simulink model "Ex6_1_1_PID2"  (R2016a)
settings: Solver=VariableStepAuto  StartTime=0.0  StopTime=20  RelTol=1e-3
libraries: simulink x1
settings Model: Creator=mende  LastModifiedBy=mende

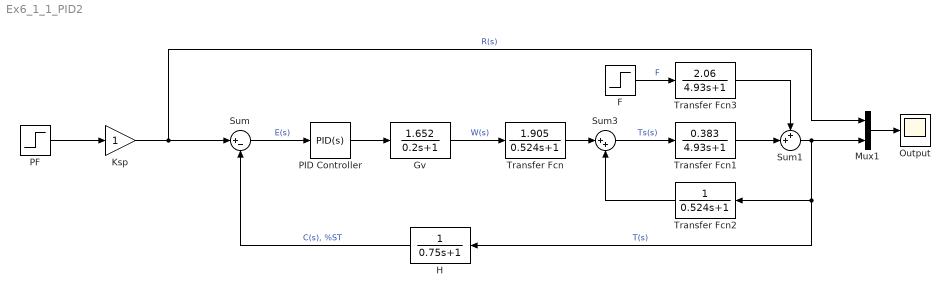
== system Ex6_1_1_PID2 ==
  F : Step  SampleTime=0
  Gv : TransferFcn  Numerator=[1.652]  Denominator=[0.2 1]
  H : TransferFcn  Denominator=[0.75 1]
  Ksp : Gain
  Mux1 : Mux  Inputs=2
  Output : Scope
  PF : Step  SampleTime=0
  PID Controller : simulink/Continuous/PID Controller  Controller=PID  TimeDomain=Continuous-time  SampleTime=-1  IntegratorMethod=Forward Euler  FilterMethod=Forward Euler  Form=Parallel  UseFilter=on  ControllerParametersSource=internal  P=6.1  I=6.1/2.3  D=6.1*0.58  N=100  InitialConditionSource=internal  InitialConditionForIntegrator=0  InitialConditionForFilter=0  ExternalReset=none  LimitOutput=off  UpperSaturationLimit=inf  LowerSaturationLimit=-inf  LinearizeAsGain=on  AntiWindupMode=none  Kb=1  TrackingMode=off  Kt=1  PParamMin=[]  PParamMax=[]  IParamMin=[]  IParamMax=[]  DParamMin=[]  DParamMax=[]  NParamMin=[]  NParamMax=[]  KbParamMin=[]  KbParamMax=[]  KtParamMin=[]  KtParamMax=[]  POutMin=[]  POutMax=[]  IOutMin=[]  IOutMax=[]  DOutMin=[]  DOutMax=[]  NOutMin=[]  NOutMax=[]  KbOutMin=[]  KbOutMax=[]  KtOutMin=[]  KtOutMax=[]  IntegratorOutMin=[]  IntegratorOutMax=[]  FilterOutMin=[]  FilterOutMax=[]  SumOutMin=[]  SumOutMax=[]  SumI1OutMin=[]  SumI1OutMax=[]  SumI2OutMin=[]  SumI2OutMax=[]  SumI3OutMin=[]  SumI3OutMax=[]  SumDOutMin=[]  SumDOutMax=[]  SaturationOutMin=[]  SaturationOutMax=[]  IntegratorContinuousStateAttributes=''  IntegratorStateMustResolveToSignalObject=off  IntegratorRTWStateStorageClass=Auto  FilterContinuousStateAttributes=''  FilterStateMustResolveToSignalObject=off  FilterRTWStateStorageClass=Auto  DifferentiatorICPrevScaledInput=0  DifferentiatorOutMin=[]  DifferentiatorOutMax=[]
  Sum : Sum  Inputs=|+-
  Sum1 : Sum  Inputs=++|
  Sum3 : Sum  Inputs=|++
  Transfer Fcn : TransferFcn  Numerator=[1.905]  Denominator=[0.524 1]
  Transfer Fcn1 : TransferFcn  Numerator=[0.383]  Denominator=[4.93 1]
  Transfer Fcn2 : TransferFcn  Denominator=[0.524 1]
  Transfer Fcn3 : TransferFcn  Numerator=[2.06]  Denominator=[4.93 1]
  wires:
  Ksp/1 -> Sum/1, Mux1/1  "R(s)"
  Gv/1 -> Transfer Fcn/1  "W(s)"
  H/1 -> Sum/2  "C(s), %ST"
  Sum1/1 -> Mux1/2, H/1, Transfer Fcn2/1  "T(s)"
  Mux1/1 -> Output/1
  PF/1 -> Ksp/1
  Transfer Fcn1/1 -> Sum1/2
  F/1 -> Transfer Fcn3/1  "F"
  Transfer Fcn3/1 -> Sum1/1
  Transfer Fcn2/1 -> Sum3/2
  Transfer Fcn/1 -> Sum3/1
  Sum3/1 -> Transfer Fcn1/1  "Ts(s)"
  PID Controller/1 -> Gv/1
  Sum/1 -> PID Controller/1  "E(s)"
